simulink model "BlinkLed"  (R2022b)
settings: Solver=VariableStepAuto  StartTime=0.0  StopTime=10.0  RelTol=1e-3
settings Model: Creator=ahmed  LastModifiedBy=ahmed

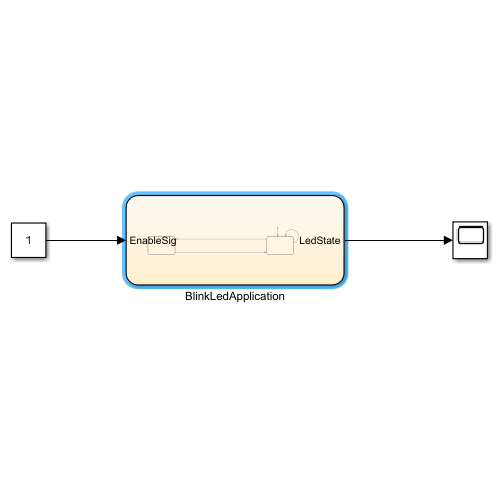
[thumbnail: Simulink's stored preview of the top-level diagram]
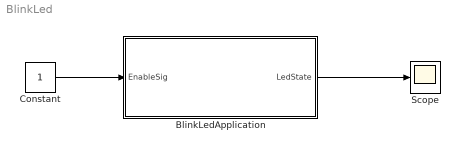
== system BlinkLed ==
  BlinkLedApplication : Stateflow chart  TreatAsAtomicUnit=on
  Constant : Constant
  Scope : Scope
  wires:
  Constant/1 -> BlinkLedApplication/1(EnableSig)
  BlinkLedApplication/1(LedState) -> Scope/1

== stateflow chart BlinkLed/BlinkLedApplication ==
  state LedOn
    en:
    LedState = 1;
  state LedOff
    en:
    LedState = 0;
  (default) -> LedOff
  LedOff -> LedOff [order 1] : [EnableSig==0]
  LedOff -> LedOn [order 2] : after(1,sec)[EnableSig == 1]
  LedOn -> LedOff : after(1,sec)
  data: LedState output; EnableSig input
